simulink model "test_bench2018b"  (Simulink 9.2)
settings: Solver=FixedStepDiscrete  StartTime=0.0  StopTime=inf  FixedStep=t_sample_s  RelTol=1e-3
values from neighbouring files (symbols this model uses):
  h_k_init = zeros(hidden_dim, num_layer)    [init.m]
  N = 4    [init.m]
  n_akt = 5    [init.m]
  t_sample_mpc_s = 1/f_sample_mpc_Hz    (= 0.2)    [init.m]
  t_sample_s = 1/f_sample_Hz    (= 0.05)    [init.m]
  u_scaler_max = double(gru_params.x_scaler_max(:,xdim+1:end))    [init.m]
  u_scaler_min = double(gru_params.x_scaler_min(:,xdim+1:end))    [init.m]
  xn_goal_ges = [xn_goal_ramp; zeros_arr]    [init.m]
  xs_goal_ges = fcn_MinMax(xn_goal_ges, y_scaler_min, y_scaler_max, [-1,1], false)    [init.m]
  y_scaler_max = double(gru_params.y_scaler_max)    [init.m]
  y_scaler_min = double(gru_params.y_scaler_min)    [init.m]
undefined symbols (not defined in the file): structParamBus
libraries: haley_test_bench_lib x23, etherlab_lib x10, dspfdesign x1
settings Model: Creator=moritz  LastModifiedBy=root  SimulationMode=external  ExtModeTrigDuration=200  ExtModeArchiveMode=auto  ExtModeArchiveFileName=measurement_data  ExtModeArchiveDirName=./results  ExtModeLogAll=off
settings DataIOCC: LimitDataPoints=off  SaveFormat=Dataset  SignalLoggingSaveFormat=Dataset  SaveOutput=off  SignalLogging=off  SaveTime=off
settings OptimizationCC: BlockReduction=off  ConditionallyExecuteInputs=off  OptimizeBlockIOStorage=off  BufferReuse=off  GlobalBufferReuse=off  ExpressionFolding=off  LocalBlockOutputs=off  LifeSpan=auto  OptimizeDataStoreBuffers=off  BusAssignmentInplaceUpdate=off
settings DebuggingCC: UnderspecifiedInitializationDetection=Simplified  MergeDetectMultiDrivingBlocksExec=error  FcnCallInpInsideContextMsg=error  StateNameClashWarn=none  SFUnexpectedBacktrackingDiag=error  SFNoUnconditionalDefaultTransitionDiag=error  SFExecutionAtInitializationDiag=warning
settings HardwareCC: ProdBitPerPointer=64  ProdBitPerSizeT=64  ProdBitPerPtrDiffT=64  ProdLargestAtomicFloat=Float  ProdIntDivRoundTo=Zero  ProdEndianess=LittleEndian  ProdWordSize=64  ProdHWDeviceType=Intel->x86-64 (Windows64)
settings ModelReferenceCC: PropagateSignalLabelsOutOfModel=on
settings RTWCC: Description=EtherLab PREEMT_RT Real-Time Target  SystemTargetFile=etherlab.tlc  TemplateMakefile=etherlab_hrt.tmf
settings CodeAppCC: StateflowObjectComments=off
settings STFCustomTargetCC: TargetLangStandard=C99 (ISO)  ModelReferenceCompliant=off  SystemTargetFile=etherlab.tlc
settings GRTTargetCC: TargetLangStandard=C99 (ISO)  ModelReferenceCompliant=off  ParMdlRefBuildCompliant=off  CompOptLevelCompliant=off  ConcurrentExecutionCompliant=off  MatFileLogging=off  CPPClassGenCompliant=off  UseToolchainInfoCompliant=off  ExtMode=on  ExtModeStaticAlloc=on  ExtModeStaticAllocSize=500000000  ExtModeMexArgs='130.75.144.164' 0 17725  RTWCAPISignals=on  RTWCAPIParams=on
settings CustomProperty: DataType=int32  Value=2
settings ConfigComp: CovMetricSettings=dwe  CovSaveCumulativeToWorkspaceVar=off  CovSaveSingleToWorkspaceVar=off  CovExternalEMLEnable=on

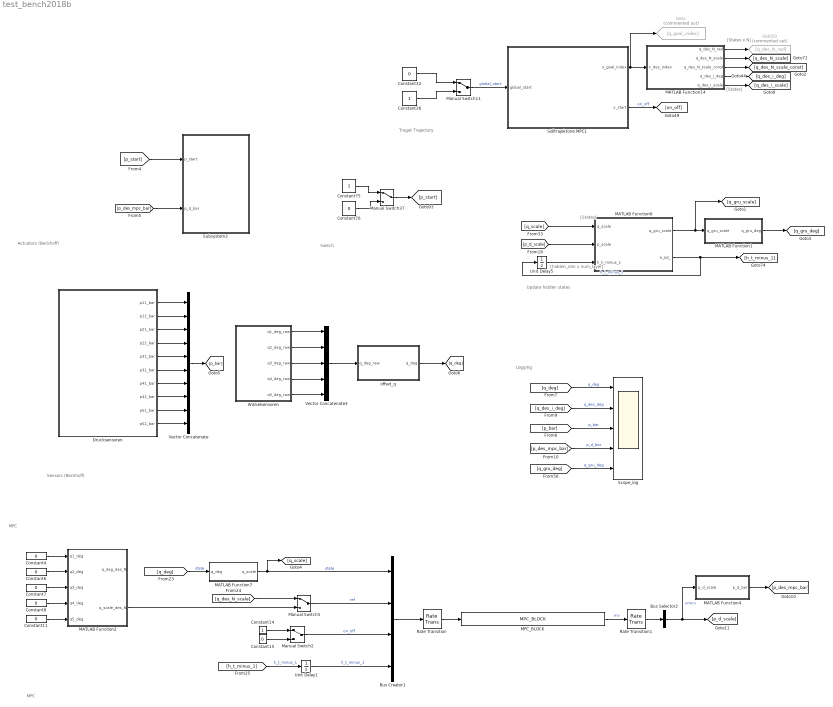
== system test_bench2018b ==
  note: MPC
  note: Sensors (Beckhoff)
  note: Actuators (Beckhoff)
  note: Switch
  note: [States x N]
  note: [States]
  note: Logging
  note: [hidden_dim x num_layer]
  note: [States]
  note: MPC
  note: Update hidden states
  note: Traget Trajectory
  Bus Creator1 : BusCreator  Inputs=4  OutDataTypeStr=Bus: MPC_IN_type
  Bus Selector2 : BusSelector  OutputSignals=mv
  Constant{4,6..8,11,76} (6 alike) : Constant  Value=0  SampleTime=t_sample_s
  Constant14 : Constant  SampleTime=t_sample_mpc_s
  Constant15 : Constant  Value=0  SampleTime=t_sample_mpc_s
  Constant32 : Constant  Value=0  SampleTime=t_sample_mpc_s
  Constant36 : Constant  SampleTime=t_sample_mpc_s
  Constant75 : Constant  SampleTime=t_sample_s
  Drucksensoren : Subsystem
  Goto : Goto  Commented=on  GotoTag=q_goal_index
  Goto50 : Goto  Commented=on  GotoTag=q_des_N_rad
  MATLAB Function1 : MATLAB Function  TreatAsAtomicUnit=on  SystemSampleTime=t_sample_mpc_s
  MATLAB Function14 : MATLAB Function  TreatAsAtomicUnit=on
  MATLAB Function2 : MATLAB Function  TreatAsAtomicUnit=on
  MATLAB Function4 : MATLAB Function  TreatAsAtomicUnit=on  SystemSampleTime=t_sample_mpc_s
  MATLAB Function6 : MATLAB Function  TreatAsAtomicUnit=on  SystemSampleTime=t_sample_mpc_s
  MATLAB Function7 : MATLAB Function  TreatAsAtomicUnit=on  SystemSampleTime=t_sample_mpc_s
  MPC_BLOCK : S-Function  FunctionName=MPC_BLOCK  Parameters=SParameter1  SFunctionDeploymentMode=off  EnableBusSupport=off  mask(Legacy Function){SFunctionSpec=void SL_io_mpc_func(MPC_IN_type u1[1], MPC_OUT_type y1[1]), SParameter1=structParamBus, ShowSpec=on}
      mask prompts: SParameter1 "P1:"; ShowSpec "Display function specification"
      mask help:
      | This block allows you to call the legacy functions specified by the following Legacy Code Tool definition:
      | def.SFunctionName = 'MPC_BLOCK';
      | def.OutputFcnSpec = 'void SL_io_mpc_func(MPC_IN_type u1[1], MPC_OUT_type y1[1])';
      | def.StartFcnSpec = 'void SL_start_mpc_func(MPC_PARAM_type p1[1])';
      | def.TerminateFcnSpec = 'void SL_terminate_mpc_func()';
      | def.HeaderFiles = {'sl_mpc.h'};
      | def.SourceFiles = {'../../src/sl_func_dummy.cpp'};
      | def.TargetLibFiles = {'libMPC_BLOCK.so', 'libcasadi.so'};
      | def.IncPaths = {'../../include/sl_function/', '/usr/local/lib/cmake/casadi'};
      | def.LibPaths = {'../build', '/usr/local/lib'};
      mask Help: <p>This block was generated automatically by the Legacy Code Tool. For detailed help on this tool, call<a href="matlab:legacy_code('help')"> legacy_code('help')</a>.</p>
      mask Callback ShowSpec:
      | if strcmp(get_param(gcbh, 'ShowSpec'), 'on')
      |   set_param(gcbh, 'MaskDisplay', sprintf('fprintf(''%s'');', get_param(gcbh, 'SFunctionSpec')));
      | else
      |   set_param(gcbh, 'MaskDisplay', sprintf('fprintf(''%s'');', get_param(gcbh, 'FunctionName')));
      | end
      mask Display: fprintf('void SL_io_mpc_func(MPC_IN_type u1[1], MPC_OUT_type y1[1])');
  Manual Switch{2,5,11,37} (4 alike) : ManualSwitch
  Rate Transition : RateTransition  OutPortSampleTime=t_sample_mpc_s
  Rate Transition1 : RateTransition  OutPortSampleTime=t_sample_s
  Scope_log : Scope  NumInputPorts=5
  Solltrajektorie MPC1 : Stateflow chart  TreatAsAtomicUnit=on
  Subsystem2 : Subsystem
  Unit Delay1 : UnitDelay  InitialCondition=h_k_init  SampleTime=t_sample_mpc_s  HasFrameUpgradeWarning=on
  Unit Delay5 : UnitDelay  InitialCondition=h_k_init  SampleTime=t_sample_mpc_s  HasFrameUpgradeWarning=on
  Vector Concatenate : Concatenate  NumInputs=10
  Vector Concatenate3 : Concatenate  NumInputs=5
  Winkelsensoren : Subsystem
  offset_q : MATLAB Function  TreatAsAtomicUnit=on
  wires:
  Drucksensoren/3("p21_bar ") -> Vector Concatenate/3
  Drucksensoren/4(p22_bar) -> Vector Concatenate/4
  Drucksensoren/1("p11_bar ") -> Vector Concatenate/1
  Drucksensoren/2(p12_bar) -> Vector Concatenate/2
  Drucksensoren/5(p31_bar) -> Vector Concatenate/5
  Drucksensoren/6(p32_bar) -> Vector Concatenate/6
  Drucksensoren/7(p41_bar) -> Vector Concatenate/7
  Drucksensoren/8(p42_bar) -> Vector Concatenate/8
  Drucksensoren/9(p51_bar) -> Vector Concatenate/9
  Drucksensoren/10(p52_bar) -> Vector Concatenate/10
  Constant76/1 -> Manual Switch37/2
  Constant75/1 -> Manual Switch37/1
  Manual Switch37/1 -> [p_start]
  Vector Concatenate/1 -> [p_bar]
  Winkelsensoren/1(q1_deg_raw) -> Vector Concatenate3/1
  Winkelsensoren/2(q2_deg_raw) -> Vector Concatenate3/2
  Winkelsensoren/3(q3_deg_raw) -> Vector Concatenate3/3
  Winkelsensoren/4(q4_deg_raw) -> Vector Concatenate3/4
  Winkelsensoren/5(q5_deg_raw) -> Vector Concatenate3/5
  Vector Concatenate3/1 -> offset_q/1(q_deg_raw)
  offset_q/1(q_deg) -> [q_deg]
  [p_start] -> Subsystem2/1(p_start)
  Constant32/1 -> Manual Switch11/1
  Manual Switch11/1 -> Solltrajektorie MPC1/1(global_start)  "global_start"
  Constant36/1 -> Manual Switch11/2
  Solltrajektorie MPC1/2(x_start) -> [on_off]  "on_off"
  Solltrajektorie MPC1/1(x_goal_index) -> MATLAB Function14/1(x_des_index), Goto/1
  MATLAB Function14/2(q_des_N_scale) -> [q_des_N_scale]
  MATLAB Function14/4(q_des_i_deg) -> [q_des_i_deg]
  MATLAB Function14/1(q_des_N_rad) -> Goto50/1
  [p_des_mpc_bar] -> Scope_log/4  "p_d_bar"
  [p_bar] -> Scope_log/3  "p_bar"
  [q_des_i_deg] -> Scope_log/2  "q_des_deg"
  [q_deg] -> Scope_log/1  "q_deg"
  MATLAB Function6/2(h_k0_) -> [h_t_minus_1], Unit Delay5/1  "h_t_minus_1"
  Unit Delay5/1 -> MATLAB Function6/3(h_k_minus_1)
  MATLAB Function6/1(q_gru_scale) -> MATLAB Function1/1(q_gru_scale), [q_gru_scale]
  [p_d_scale] -> MATLAB Function6/2(p_scale)
  MATLAB Function1/1(q_gru_deg) -> [q_gru_deg]
  MPC_BLOCK/1 -> Rate Transition1/1  "mv"
  Bus Selector2/1 -> [p_d_scale], MATLAB Function4/1(p_d_scale)  "<mv>"
  Manual Switch5/1 -> Bus Creator1/2  "ref"
  Manual Switch2/1 -> Bus Creator1/3  "on_off"
  MATLAB Function4/1(p_d_bar) -> [p_des_mpc_bar]
  Constant14/1 -> Manual Switch2/1
  Constant15/1 -> Manual Switch2/2
  [p_des_mpc_bar] -> Subsystem2/2(p_d_bar)
  Bus Creator1/1 -> Rate Transition/1
  [h_t_minus_1] -> Unit Delay1/1  "h_t_minus_1"
  Unit Delay1/1 -> Bus Creator1/4  "h_t_minus_1"
  [q_des_N_scale] -> Manual Switch5/1
  [q_deg] -> MATLAB Function7/1(q_deg)  "state"
  MATLAB Function7/1(q_scale) -> [q_scale], Bus Creator1/1  "state"
  MATLAB Function14/5(q_des_i_scale) -> [q_des_i_scale]
  MATLAB Function14/3(q_des_N_scale_const) -> [q_des_N_scale_const]
  Constant4/1 -> MATLAB Function2/1(q1_deg)
  Constant6/1 -> MATLAB Function2/2(q2_deg)
  Constant7/1 -> MATLAB Function2/3(q3_deg)
  Constant8/1 -> MATLAB Function2/4(q4_deg)
  Constant11/1 -> MATLAB Function2/5(q5_deg)
  MATLAB Function2/2(q_scale_des_N) -> Manual Switch5/2
  [q_scale] -> MATLAB Function6/1(q_scale)
  Rate Transition/1 -> MPC_BLOCK/1
  Rate Transition1/1 -> Bus Selector2/1
  [q_gru_deg] -> Scope_log/5  "q_gru_deg"

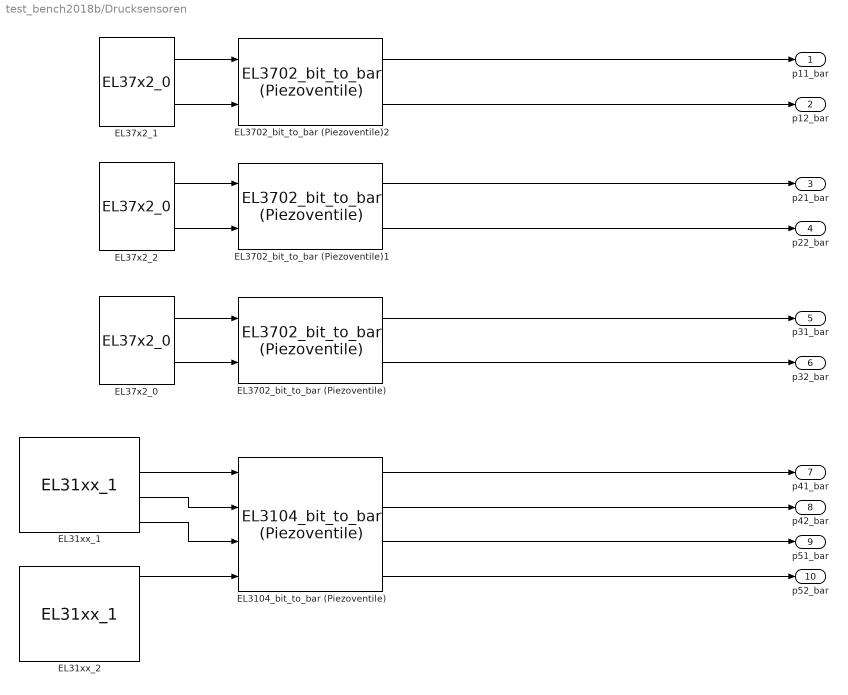
== system test_bench2018b/Drucksensoren ==
  EL3104_bit_to_bar (Piezoventile) : haley_test_bench_lib/EL3104_bit_to_bar (Piezoventile)  SystemSampleTime=-1
  EL31xx_1 : etherlab_lib/EtherCAT/Beckhoff/EL31xx_1  master=0  index=8  model=EL3104  revision=[203436114 1179648]  vector=off  status=off  filter=Off  gain=[]  offset=[]  tau=[]  tsample=t_sample_s  debug=0  dc_mode=Free Run/SM-Synchron  dc_assign_activate=hex2dec('700')  dc_cycle0=[]  dc_cycle0_factor=[]  dc_shift0=[]  dc_shift0_factor=[]  dc_shift0_input=off  dc_cycle1=[]  dc_cycle1_factor=[]  dc_shift1=[]  dc_shift1_factor=[]
      settings: AttributesFormatString=|
      | EL3104
      | M:0 Idx:8
  EL31xx_2 : etherlab_lib/EtherCAT/Beckhoff/EL31xx_1  master=0  index=9  model=EL3104  revision=[203436114 1179648]  vector=off  status=off  filter=Off  gain=[]  offset=[]  tau=[]  tsample=t_sample_s  debug=0  dc_mode=Free Run/SM-Synchron  dc_assign_activate=hex2dec('700')  dc_cycle0=[]  dc_cycle0_factor=[]  dc_shift0=[]  dc_shift0_factor=[]  dc_shift0_input=off  dc_cycle1=[]  dc_cycle1_factor=[]  dc_shift1=[]  dc_shift1_factor=[]
      settings: AttributesFormatString=|
      | EL3104
      | M:0 Idx:9
  EL3702_bit_to_bar (Piezoventile) : haley_test_bench_lib/EL3702_bit_to_bar (Piezoventile)  SystemSampleTime=-1
  EL3702_bit_to_bar (Piezoventile)1 : haley_test_bench_lib/EL3702_bit_to_bar (Piezoventile)  SystemSampleTime=-1
  EL3702_bit_to_bar (Piezoventile)2 : haley_test_bench_lib/EL3702_bit_to_bar (Piezoventile)  SystemSampleTime=-1
  EL37x2_0 : etherlab_lib/EtherCAT/Beckhoff/EL37x2_0  master=0  index=5  model=EL3702  revision=[242626642 131072]  one_ch=off  scale=[]  offset=[]  tsample=t_sample_s  debug=0  dc_mode=1  dc_assign_activate=hex2dec('730')  dc_cycle0=0  dc_cycle0_factor="-10     % 10-times OS"  dc_shift0=-10000  dc_shift0_factor=1  dc_shift0_input=off  dc_cycle1=0  dc_cycle1_factor=-1  dc_shift1=0  dc_shift1_factor=0
  EL37x2_1 : etherlab_lib/EtherCAT/Beckhoff/EL37x2_0  master=0  index=3  model=EL3702  revision=[242626642 131072]  one_ch=off  scale=[]  offset=[]  tsample=t_sample_s  debug=0  dc_mode=1  dc_assign_activate=hex2dec('730')  dc_cycle0=0  dc_cycle0_factor="-10     % 10-times OS"  dc_shift0=-10000  dc_shift0_factor=1  dc_shift0_input=off  dc_cycle1=0  dc_cycle1_factor=-1  dc_shift1=0  dc_shift1_factor=0
  EL37x2_2 : etherlab_lib/EtherCAT/Beckhoff/EL37x2_0  master=0  index=4  model=EL3702  revision=[242626642 131072]  one_ch=off  scale=[]  offset=[]  tsample=t_sample_s  debug=0  dc_mode=1  dc_assign_activate=hex2dec('730')  dc_cycle0=0  dc_cycle0_factor="-10     % 10-times OS"  dc_shift0=-10000  dc_shift0_factor=1  dc_shift0_input=off  dc_cycle1=0  dc_cycle1_factor=-1  dc_shift1=0  dc_shift1_factor=0
  "p11_bar " : Outport  VectorParamsAs1DForOutWhenUnconnected=off
  p12_bar : Outport  Port=2  VectorParamsAs1DForOutWhenUnconnected=off
  "p21_bar " : Outport  Port=3  VectorParamsAs1DForOutWhenUnconnected=off
  p22_bar : Outport  Port=4  VectorParamsAs1DForOutWhenUnconnected=off
  p31_bar : Outport  Port=5  VectorParamsAs1DForOutWhenUnconnected=off
  p32_bar : Outport  Port=6  VectorParamsAs1DForOutWhenUnconnected=off
  p41_bar : Outport  Port=7  VectorParamsAs1DForOutWhenUnconnected=off
  p42_bar : Outport  Port=8  VectorParamsAs1DForOutWhenUnconnected=off
  p51_bar : Outport  Port=9  VectorParamsAs1DForOutWhenUnconnected=off
  p52_bar : Outport  Port=10  VectorParamsAs1DForOutWhenUnconnected=off
  wires:
  EL37x2_0/1 -> EL3702_bit_to_bar (Piezoventile)/1
  EL3702_bit_to_bar (Piezoventile)/2 -> p32_bar/1
  EL3702_bit_to_bar (Piezoventile)/1 -> p31_bar/1
  EL37x2_0/2 -> EL3702_bit_to_bar (Piezoventile)/2
  EL37x2_1/2 -> EL3702_bit_to_bar (Piezoventile)2/2
  EL37x2_1/1 -> EL3702_bit_to_bar (Piezoventile)2/1
  EL3702_bit_to_bar (Piezoventile)1/2 -> p22_bar/1
  EL37x2_2/2 -> EL3702_bit_to_bar (Piezoventile)1/2
  EL37x2_2/1 -> EL3702_bit_to_bar (Piezoventile)1/1
  EL3702_bit_to_bar (Piezoventile)1/1 -> "p21_bar "/1
  EL3702_bit_to_bar (Piezoventile)2/1 -> "p11_bar "/1
  EL3702_bit_to_bar (Piezoventile)2/2 -> p12_bar/1
  EL3104_bit_to_bar (Piezoventile)/2 -> p42_bar/1
  EL3104_bit_to_bar (Piezoventile)/1 -> p41_bar/1
  EL3104_bit_to_bar (Piezoventile)/4 -> p52_bar/1
  EL3104_bit_to_bar (Piezoventile)/3 -> p51_bar/1
  EL31xx_1/2 -> EL3104_bit_to_bar (Piezoventile)/1
  EL31xx_1/3 -> EL3104_bit_to_bar (Piezoventile)/2
  EL31xx_1/4 -> EL3104_bit_to_bar (Piezoventile)/3
  EL31xx_2/1 -> EL3104_bit_to_bar (Piezoventile)/4

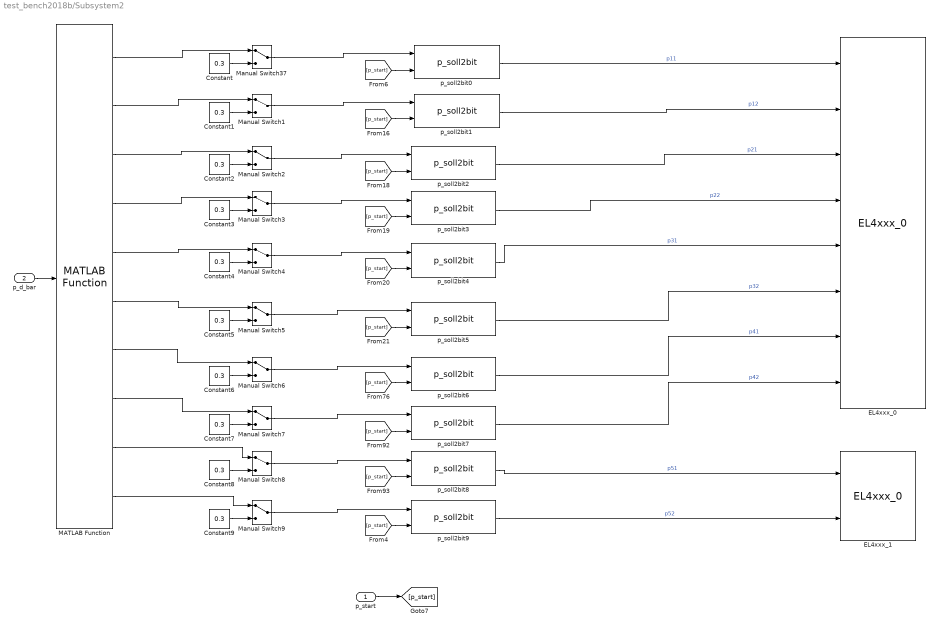
== system test_bench2018b/Subsystem2 ==
  p_start : Inport
  p_d_bar : Inport  Port=2
  Constant{,1..9} (10 alike) : Constant  Value=0.3  SampleTime=t_sample_s
  EL4xxx_0 : etherlab_lib/EtherCAT/Beckhoff/EL4xxx_0  master=0  index=10  model=EL4008  revision=[262680658 1245184]  vector=off  scale=[]  tsample=t_sample_s  debug=0  dc_mode=Free Run  dc_assign_activate=hex2dec('700')  dc_cycle0=0  dc_cycle0_factor=1  dc_shift0=0  dc_shift0_factor=0  dc_shift0_input=off  dc_cycle1=0  dc_cycle1_factor=1  dc_shift1=10000  dc_shift1_factor=0
  EL4xxx_1 : etherlab_lib/EtherCAT/Beckhoff/EL4xxx_0  master=0  index=11  model=EL4102  revision=[268841042 66715648]  vector=off  scale=[]  tsample=t_sample_s  debug=0  dc_mode=Free Run  dc_assign_activate=hex2dec('700')  dc_cycle0=0  dc_cycle0_factor=1  dc_shift0=0  dc_shift0_factor=0  dc_shift0_input=off  dc_cycle1=0  dc_cycle1_factor=1  dc_shift1=10000  dc_shift1_factor=0
  MATLAB Function : haley_test_bench_lib/MATLAB Function  SystemSampleTime=-1
  Manual Switch{1..9,37} (10 alike) : ManualSwitch
  p_soll2bit{0..9} (10 alike) : haley_test_bench_lib/p_soll2bit  SystemSampleTime=-1
  wires:
  [p_start] -> p_soll2bit3/2
  p_soll2bit9/1 -> EL4xxx_1/2  "p52"
  p_soll2bit7/1 -> EL4xxx_0/8  "p42"
  p_soll2bit5/1 -> EL4xxx_0/6  "p32"
  [p_start] -> p_soll2bit9/2
  [p_start] -> p_soll2bit6/2
  p_soll2bit6/1 -> EL4xxx_0/7  "p41"
  [p_start] -> p_soll2bit8/2
  p_soll2bit8/1 -> EL4xxx_1/1  "p51"
  [p_start] -> p_soll2bit2/2
  p_soll2bit4/1 -> EL4xxx_0/5  "p31"
  p_soll2bit3/1 -> EL4xxx_0/4  "p22"
  MATLAB Function/4 -> Manual Switch3/1
  [p_start] -> p_soll2bit1/2
  MATLAB Function/5 -> Manual Switch4/1
  p_soll2bit1/1 -> EL4xxx_0/2  "p12"
  p_soll2bit2/1 -> EL4xxx_0/3  "p21"
  [p_start] -> p_soll2bit7/2
  MATLAB Function/1 -> Manual Switch37/1
  p_start/1 -> [p_start]
  [p_start] -> p_soll2bit4/2
  MATLAB Function/9 -> Manual Switch8/1
  [p_start] -> p_soll2bit5/2
  [p_start] -> p_soll2bit0/2
  MATLAB Function/8 -> Manual Switch7/1
  MATLAB Function/7 -> Manual Switch6/1
  MATLAB Function/2 -> Manual Switch1/1
  MATLAB Function/10 -> Manual Switch9/1
  MATLAB Function/6 -> Manual Switch5/1
  MATLAB Function/3 -> Manual Switch2/1
  p_d_bar/1 -> MATLAB Function/1
  Manual Switch37/1 -> p_soll2bit0/1
  Manual Switch1/1 -> p_soll2bit1/1
  Manual Switch2/1 -> p_soll2bit2/1
  Manual Switch3/1 -> p_soll2bit3/1
  Manual Switch4/1 -> p_soll2bit4/1
  Manual Switch5/1 -> p_soll2bit5/1
  Manual Switch6/1 -> p_soll2bit6/1
  Manual Switch7/1 -> p_soll2bit7/1
  Manual Switch8/1 -> p_soll2bit8/1
  Constant/1 -> Manual Switch37/2
  Constant1/1 -> Manual Switch1/2
  Constant2/1 -> Manual Switch2/2
  Constant3/1 -> Manual Switch3/2
  Constant4/1 -> Manual Switch4/2
  Constant5/1 -> Manual Switch5/2
  Constant6/1 -> Manual Switch6/2
  Constant7/1 -> Manual Switch7/2
  Constant8/1 -> Manual Switch8/2
  Constant9/1 -> Manual Switch9/2
  Manual Switch9/1 -> p_soll2bit9/1
  p_soll2bit0/1 -> EL4xxx_0/1  "p11"

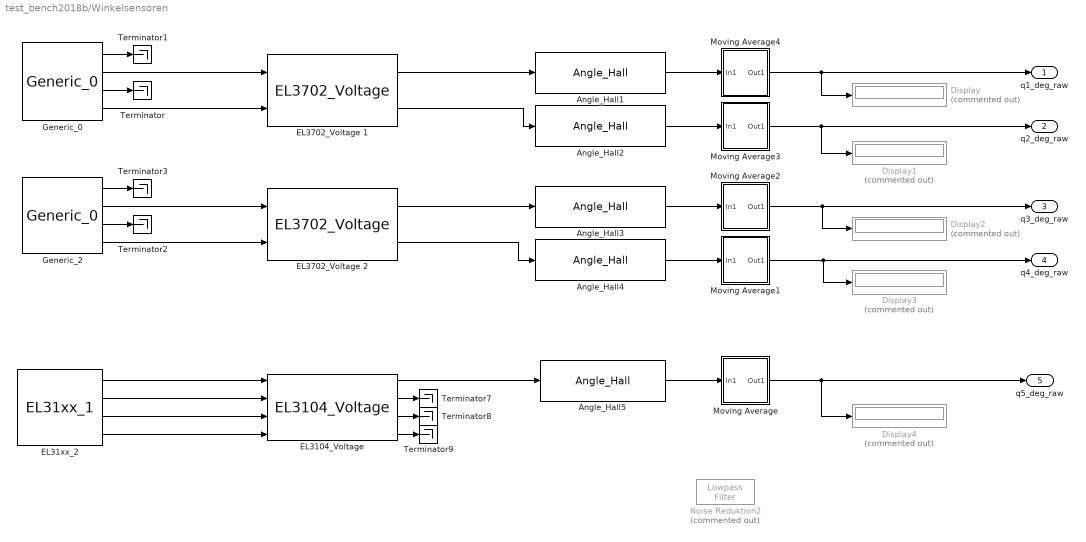
== system test_bench2018b/Winkelsensoren ==
  Angle_Hall{1..5} (5 alike) : haley_test_bench_lib/Angle_Hall  SystemSampleTime=-1
  Display{,1..4} (5 alike) : Display  Commented=on
  EL3104_Voltage : haley_test_bench_lib/EL3104_Voltage  SystemSampleTime=-1
  EL31xx_2 : etherlab_lib/EtherCAT/Beckhoff/EL31xx_1  master=0  index=8  model=EL3104  revision=[203436114 1179648]  vector=off  status=off  filter=Off  gain=[]  offset=[]  tau=[]  tsample=t_sample_s  debug=0  dc_mode=Free Run/SM-Synchron  dc_assign_activate=hex2dec('700')  dc_cycle0=[]  dc_cycle0_factor=[]  dc_shift0=[]  dc_shift0_factor=[]  dc_shift0_input=off  dc_cycle1=[]  dc_cycle1_factor=[]  dc_shift1=[]  dc_shift1_factor=[]
      settings: AttributesFormatString=|
      | EL3104
      | M:0 Idx:8
  EL3702_Voltage 1 : haley_test_bench_lib/EL3702_Voltage  SystemSampleTime=-1
  EL3702_Voltage 2 : haley_test_bench_lib/EL3702_Voltage  SystemSampleTime=-1
  Generic_0 : etherlab_lib/EtherCAT/Generic_0  master=0  index=6  rv=slave_el3102  param=[]  tsample=t_sample_s  debug=0
  Generic_2 : etherlab_lib/EtherCAT/Generic_0  master=0  index=7  rv=slave_el3102  param=[]  tsample=t_sample_s  debug=0
  Moving Average : Subsystem  Description=Replaced Block  InitFcn=error('This block was designed with a newer version of Simulink. Unfortunately, your Simulink version does not support these features.')  mask(Replaced Block){}
      mask help: This block has been replaced with an empty subsystem because it used functionality that is unavailable in Simulink R2018b.
      mask Display: fprintf('Replaced: %s\n','Moving Statistics with Overlap Length not equal to Window Length - 1 (supported from R2022b).')
  Moving Average1 : Subsystem  Description=Replaced Block  InitFcn=error('This block was designed with a newer version of Simulink. Unfortunately, your Simulink version does not support these features.')  mask(Replaced Block){}
      mask help: This block has been replaced with an empty subsystem because it used functionality that is unavailable in Simulink R2018b.
      mask Display: fprintf('Replaced: %s\n','Moving Statistics with Overlap Length not equal to Window Length - 1 (supported from R2022b).')
  Moving Average2 : Subsystem  Description=Replaced Block  InitFcn=error('This block was designed with a newer version of Simulink. Unfortunately, your Simulink version does not support these features.')  mask(Replaced Block){}
      mask help: This block has been replaced with an empty subsystem because it used functionality that is unavailable in Simulink R2018b.
      mask Display: fprintf('Replaced: %s\n','Moving Statistics with Overlap Length not equal to Window Length - 1 (supported from R2022b).')
  Moving Average3 : Subsystem  Description=Replaced Block  InitFcn=error('This block was designed with a newer version of Simulink. Unfortunately, your Simulink version does not support these features.')  mask(Replaced Block){}
      mask help: This block has been replaced with an empty subsystem because it used functionality that is unavailable in Simulink R2018b.
      mask Display: fprintf('Replaced: %s\n','Moving Statistics with Overlap Length not equal to Window Length - 1 (supported from R2022b).')
  Moving Average4 : Subsystem  Description=Replaced Block  InitFcn=error('This block was designed with a newer version of Simulink. Unfortunately, your Simulink version does not support these features.')  mask(Replaced Block){}
      mask help: This block has been replaced with an empty subsystem because it used functionality that is unavailable in Simulink R2018b.
      mask Display: fprintf('Replaced: %s\n','Moving Statistics with Overlap Length not equal to Window Length - 1 (supported from R2022b).')
  Noise Reduktion2 : dspfdesign/Lowpass Filter  Commented=on  FilterType=FIR  DesignForMinimumOrder=on  FilterOrder=50  PassbandFrequency=passband_freq_Hz  StopbandFrequency=stopband_freq_Hz  PassbandRipple=passband_ripple_dB  StopbandAttenuation=stopband_atten_dB  SampleRate=1/t_sample_s  SimulateUsing=Interpreted execution  roundingMode=Floor  coeffsDataTypeStr=fixdt(1,16)  InheritSampleRate=off
  Terminator{,1..3,7..9} (7 alike) : Terminator
  q1_deg_raw : Outport  VectorParamsAs1DForOutWhenUnconnected=off
  q2_deg_raw : Outport  Port=2  VectorParamsAs1DForOutWhenUnconnected=off
  q3_deg_raw : Outport  Port=3  VectorParamsAs1DForOutWhenUnconnected=off
  q4_deg_raw : Outport  Port=4  VectorParamsAs1DForOutWhenUnconnected=off
  q5_deg_raw : Outport  Port=5  VectorParamsAs1DForOutWhenUnconnected=off
  wires:
  EL3702_Voltage 1/1 -> Angle_Hall1/1
  Angle_Hall1/1 -> Moving Average4/1(In1)
  Moving Average4/1(Out1) -> q1_deg_raw/1, Display/1
  Moving Average1/1(Out1) -> Display3/1, q4_deg_raw/1
  Generic_0/4 -> EL3702_Voltage 1/2
  EL3702_Voltage 2/1 -> Angle_Hall3/1
  Generic_2/4 -> EL3702_Voltage 2/2
  Moving Average3/1(Out1) -> Display1/1, q2_deg_raw/1
  Angle_Hall3/1 -> Moving Average2/1(In1)
  EL31xx_2/1 -> EL3104_Voltage/1
  Moving Average/1(Out1) -> q5_deg_raw/1, Display4/1
  EL3104_Voltage/3 -> Terminator8/1
  Angle_Hall4/1 -> Moving Average1/1(In1)
  Generic_0/3 -> Terminator/1
  Generic_0/2 -> EL3702_Voltage 1/1
  EL3702_Voltage 1/2 -> Angle_Hall2/1
  Angle_Hall5/1 -> Moving Average/1(In1)
  Generic_2/3 -> Terminator2/1
  Moving Average2/1(Out1) -> Display2/1, q3_deg_raw/1
  EL3104_Voltage/2 -> Terminator7/1
  EL3104_Voltage/1 -> Angle_Hall5/1
  EL3702_Voltage 2/2 -> Angle_Hall4/1
  Generic_2/1 -> Terminator3/1
  Generic_0/1 -> Terminator1/1
  Angle_Hall2/1 -> Moving Average3/1(In1)
  Generic_2/2 -> EL3702_Voltage 2/1
  EL3104_Voltage/4 -> Terminator9/1
  EL31xx_2/2 -> EL3104_Voltage/2
  EL31xx_2/3 -> EL3104_Voltage/3
  EL31xx_2/4 -> EL3104_Voltage/4

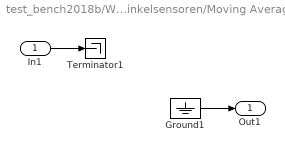
== system test_bench2018b/Winkelsensoren/Moving Average ==
  In1 : Inport
  Ground1 : Ground
  Terminator1 : Terminator
  Out1 : Outport
  wires:
  Ground1/1 -> Out1/1
  In1/1 -> Terminator1/1

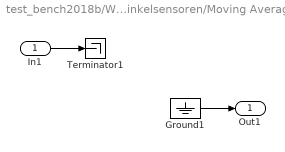
== system test_bench2018b/Winkelsensoren/Moving Average1 ==
  In1 : Inport
  Ground1 : Ground
  Terminator1 : Terminator
  Out1 : Outport
  wires:
  Ground1/1 -> Out1/1
  In1/1 -> Terminator1/1

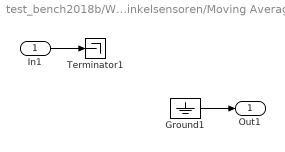
== system test_bench2018b/Winkelsensoren/Moving Average2 ==
  In1 : Inport
  Ground1 : Ground
  Terminator1 : Terminator
  Out1 : Outport
  wires:
  Ground1/1 -> Out1/1
  In1/1 -> Terminator1/1

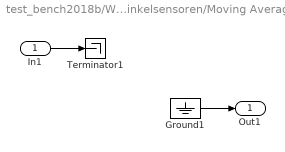
== system test_bench2018b/Winkelsensoren/Moving Average3 ==
  In1 : Inport
  Ground1 : Ground
  Terminator1 : Terminator
  Out1 : Outport
  wires:
  Ground1/1 -> Out1/1
  In1/1 -> Terminator1/1

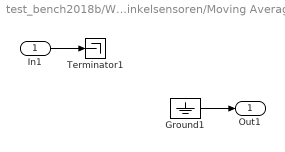
== system test_bench2018b/Winkelsensoren/Moving Average4 ==
  In1 : Inport
  Ground1 : Ground
  Terminator1 : Terminator
  Out1 : Outport
  wires:
  Ground1/1 -> Out1/1
  In1/1 -> Terminator1/1

== matlab function MATLAB Function1 ==
  data: q_gru_scale input double; q_gru_deg output double; y_scaler_max parameter double; y_scaler_min parameter double
function q_gru_deg  = scale_inverse(q_gru_scale, y_scaler_max, y_scaler_min)

    max = 1;
    min = -1;
   
    data_std = zeros(5,1);
    data = zeros(5,1);
       
    for i = 1:5
        % inverse Min-Max Transformation
        data_std(i) = (q_gru_scale(i) - min) / (max - min);
        data(i) = data_std(i) .* (y_scaler_max(i) - y_scaler_min(i)) + y_scaler_min(i);
    end
    
    q_gru_rad = reshape(double(data),5,1);
    q_gru_deg = rad2deg(q_gru_rad);
    
end

== matlab function MATLAB Function4 ==
  data: p_d_scale input double; p_d_bar output double; u_scaler_max parameter double; u_scaler_min parameter double
function p_d_bar  = scale(p_d_scale, u_scaler_max, u_scaler_min)
    max = 1;
    min = -1;
    n_akt = 5;
    data_std = zeros(2*n_akt,1);
    data = zeros(2*n_akt,1);
       
    for i = 1:2*n_akt
        % inverse Min-Max Transformation
        data_std(i) = (p_d_scale(i) - min) / (max - min);
        data(i) = data_std(i) .* (u_scaler_max(i) - u_scaler_min(i)) + u_scaler_min(i);
    end
    
    p_d_Pa = reshape(double(data),2*n_akt,1);
    p_d_bar = p_d_Pa / 1e5;
    
end

== matlab function MATLAB Function2 ==
  data: q1_deg input double; q_deg_des_N output double; q2_deg input double; q3_deg input double; q4_deg input double; q5_deg input double; q_scale_des_N output double; y_scaler_min parameter double; y_scaler_max parameter double
function [q_deg_des_N, q_scale_des_N] = qscalar2vec(q1_deg,q2_deg,q3_deg,q4_deg,q5_deg, y_scaler_min, y_scaler_max)
    
    N = 4; % Prädiktionshorizont, übergabe als variable hat nicht funktionert
    x = N+1;

    q_deg_des_i = zeros(5,1);
    q_deg_des_N = zeros(5,x);
    q_scale_des_N = zeros(5,x);

    q_deg_des_i(1) = q1_deg;
    q_deg_des_i(2) = q2_deg;
    q_deg_des_i(3) = q3_deg;
    q_deg_des_i(4) = q4_deg;
    q_deg_des_i(5) = q5_deg;
    
    %% Skalieren
    q_rad = deg2rad(q_deg_des_i);
    % Bereich auf den Transformiert wird
    max = 1;
    min = -1;
    
    features = size(q_rad,1);
    data_std = zeros(size(q_rad));
    data_scaled = zeros(size(q_rad));
    
    for i = 1:features
        % Min-Max Transformation
        data_std(i) = (q_rad(i) - y_scaler_min(i)) ./ (y_scaler_max(i) - y_scaler_min(i));
        data_scaled(i) = data_std(i) * (max - min) + min;
    end
        
    data_scaled = double(data_scaled); % nlmpc braucht double Format und nicht single
    
    q_scale_des_N_ = repmat(reshape(data_scaled,5,1),1,x);
    q_deg_des_N_ = repmat(reshape(q_deg_des_i,5,1),1,x);
    
    for i=1:5 % n_akt
        for j=1:x % N
            q_scale_des_N(i,j) = q_scale_des_N_(i,j);
            q_deg_des_N(i,j) = q_deg_des_N_(i,j);
        end
    end
end

== matlab function MATLAB Function7 ==
  data: q_deg input double; q_scale output double; y_scaler_max parameter double; y_scaler_min parameter double
function q_scale  = scale(q_deg, y_scaler_max, y_scaler_min)

    q_rad = deg2rad(q_deg);
    
    % Bereich auf den Transformiert wird
    max = 1;
    min = -1;
    
    features = size(q_rad,1);
    data_std = zeros(size(q_rad));
    data_scaled = zeros(size(q_rad));
    
    for i = 1:features
        % Min-Max Transformation
        data_std(i) = (q_rad(i) - y_scaler_min(i)) ./ (y_scaler_max(i) - y_scaler_min(i));
        data_scaled(i) = data_std(i) * (max - min) + min;
    end
    
    data_scaled = double(data_scaled); % nlmpc braucht double Format und nicht single
    q_scale = reshape(data_scaled,5,1);
    
end

== matlab function MATLAB Function14 ==
  data: x_des_index input double; q_des_N_rad output double; q_des_N_scale output double; q_des_N_scale_const output double; xn_goal_ges parameter double; xs_goal_ges parameter double; N parameter double; n_akt parameter double; q_des_i_deg output double; q_des_i_scale output double
function [q_des_N_rad, q_des_N_scale, q_des_N_scale_const, q_des_i_deg, q_des_i_scale] = trajectory(x_des_index, xn_goal_ges, xs_goal_ges, N, n_akt)
    
    %% Definition Dimensionen
    q_des_N_rad = zeros(n_akt,N+1);
    q_des_N_scale = zeros(n_akt,N+1);
    q_des_N_scale_const = zeros(n_akt,N+1);
    
    %%
    q_des_N_rad_ = xn_goal_ges(x_des_index:(x_des_index+N),:);
    q_des_N_rad_ = q_des_N_rad_';
    q_des_i_deg_ =  xn_goal_ges(x_des_index,:);
    q_des_i_deg_ = rad2deg(q_des_i_deg_);
    q_des_i_deg = reshape(q_des_i_deg_,n_akt,1);
    
    q_des_N_scale_ = xs_goal_ges(x_des_index:(x_des_index+N),:);
    q_des_N_scale_ = q_des_N_scale_';
    q_des_i_scale_ =  xs_goal_ges(x_des_index,:);
    q_des_i_scale = reshape(q_des_i_scale_,n_akt,1);
    q_des_N_scale_const_ = repmat(q_des_i_scale,1,N+1);
    
    % Outputs schreiben
    for i = 1:n_akt % führt zu Fehlermeldung wenn die Werte nicht einzeln übergeben werden
        for j = 1:N+1
            q_des_N_rad(i,j) = q_des_N_rad_(i,j);
            q_des_N_scale(i,j) = q_des_N_scale_(i,j);
            q_des_N_scale_const(i,j) = q_des_N_scale_const_(i,j);
        end
    end

end

== stateflow chart Solltrajektorie MPC1 ==
  settings: executeAtInitialization=1
  state Prepare
    counter=1;
    x_start=0;
    x_goal_index = counter;
  state Start_Trajektorie
    x_start=1;
    x_goal_index = counter;
  state Start
    x_start=0;
  (default) -> Prepare
  Start_Trajektorie -> Prepare [order 2] : [counter >= length(xn_goal_ges)-N]
  Start_Trajektorie -> Prepare [order 1] : [global_start==0]
  Start -> Prepare [order 1] : [global_start==0]
  Prepare -> Start : [global_start==1]
  Start -> Start_Trajektorie [order 2] : after(0.5,sec)
  Start_Trajektorie -> Start_Trajektorie [order 3] : [counter<length(xn_goal_ges)-N]{counter=counter+1;}
  data: global_start input double; counter local double; N parameter double; xn_goal_ges parameter double; x_goal_index output single; x_start output double

== matlab function MATLAB Function6 ==
  data: q_scale input double; p_scale input double; q_gru_scale output double; h_k_minus_1 input double; h_k0_ output double; gru_weights parameter double
function [q_gru_scale, h_k0_] = GRU_1_layer(q_scale, p_scale, h_k_minus_1, gru_weights)

    p_scale = reshape(p_scale,10,1);
    q_scale = reshape(q_scale,5,1);
    x_k = vertcat(q_scale, p_scale);

    % Dimensionen
    q_gru_scale = zeros(5,1);
    h_k0_ = zeros(size(h_k_minus_1));
    h_k0_minus_1 = h_k_minus_1(:,1); % h_t0_minus_1 muss Dimension [hidden_dim, 1] haben % Layer 1

    % Hiddenlayer 0 von GRU
    r_k0 = sigmoid(gru_weights.w_ir_l0 * x_k + gru_weights.b_ir_l0' + gru_weights.w_hr_l0 * h_k0_minus_1 + gru_weights.b_hr_l0'); % Reset Gate
    z_k0 = sigmoid(gru_weights.w_iz_l0 * x_k + gru_weights.b_iz_l0' + gru_weights.w_hz_l0 * h_k0_minus_1 + gru_weights.b_hz_l0'); % Update Gate
    n_k0 = tanh(gru_weights.w_in_l0 * x_k + gru_weights.b_in_l0' + r_k0 .* (gru_weights.w_hn_l0 * h_k0_minus_1 + gru_weights.b_hn_l0')); % New Gate
    h_k0 = (1 - z_k0) .* n_k0 + z_k0 .* h_k0_minus_1;
    
    % Lineares Output Layer
    x_k_plus_1 = gru_weights.weight_linout * h_k0 + gru_weights.bias_linout';

    % Werte an Output übergeben
    for i = 1:5
        q_gru_scale(i) = x_k_plus_1(i);
    end
    q_gru_scale = reshape(q_gru_scale,5,1);
    
    for i = 1:size(h_k0,1)
        for j = 1:size(h_k0,2)
            h_k0_(i,j) = h_k0(i,j);
        end
    end
end

function out = sigmoid(x)
% Funktion wendet die Sigmoid-Funktion auf den Input-Vektor x an
out = 1 ./ (1 + exp(-x));
end

== matlab function offset_q ==
  data: q_deg_raw input double; q_deg output double; offset_q parameter double
function q_deg = subtract_offset(q_deg_raw,offset_q)

q_deg = q_deg_raw-offset_q';
